simulink model "pmsm_ctrl"  (R2018a)
settings: Solver=FixedStepDiscrete  StartTime=0.0  StopTime=3  FixedStep=FastTsample / 10.  RelTol=1e-3  EnableMultiTasking=on
model workspace (MATLAB code in the model file):
  | cmdLim = Simulink.Parameter;
  | cmdLim.Value = 15;
  | cmdLim.Description = 'Limit for controlling the maximum surface command angle.';
  | cmdLim.Min = 0;
  | cmdLim.Max = 90;
  | cmdLim.DocUnits = 'deg';
  | 
  | dispGain = Simulink.Parameter;
  | dispGain.Value = 0.75;
  | dispGain.Description = 'Gain applied to the displacement error.';
  | dispGain.Min = 0;
  | dispGain.Max = [];
  | dispGain.DocUnits = 'deg/sec/deg';
  | 
  | dispLim = Simulink.Parameter;
  | dispLim.Value = 30;
  | dispLim.Description = 'Limit for controlling the maximum commanded angle.';
  | dispLim.Min = 0;
  | dispLim.Max = 180;
  | dispLim.DocUnits = 'deg';
  | 
  | intGain = Simulink.Parameter;
  | intGain.Value = 0.5;
  | intGain.Description = 'Gain applied to the integral error.';
  | intGain.Min = 0;
  | intGain.Max = [];
  | intGain.DocUnits = 'deg/sec/deg/sec';
  | 
  | intLim = Simulink.Parameter;
  | intLim.Value = 5;
  | intLim.Description = 'Limit for controlling the maximum commanded angle.';
  | intLim.Min = 0;
  | intLim.Max = 90;
  | intLim.DocUnits = 'deg';
  | 
  | rateGain = Simulink.Parameter;
  | rateGain.Value = 2;
  | rateGain.Description = 'Gain applied to the rate error.';
  | rateGain.Min = 0;
  | rateGain.Max = [];
  | rateGain.DocUnits = 'deg/deg/sec';
  | 
  | rateLim = Simulink.Parameter;
  | rateLim.Value = 6;
  | rateLim.Description = 'Limit for controlling the maximum commanded angle.';
  | rateLim.Min = 0;
  | rateLim.Max = 180;
  | rateLim.DocUnits = 'deg/sec';
  | 
  | hdgGain = Simulink.Parameter;
  | hdgGain.Value = 0.015;
undefined symbols (not defined in the file): CalMgrSt_T, Cfg_AnglOfsCalPwmDuty, Cfg_AutoCalEnbl, Cfg_EnblDynComp, Cfg_EnblTrajPlan, Cfg_EncCnts, Cfg_EncOfsCalPwmDuty, Cfg_IfbkCtrlBW, Cfg_IndCalPwmDuty, Cfg_Ls, Cfg_MFlux, Cfg_MtrJm, Cfg_MtrKf, Cfg_MtrKtrq, Cfg_PolePairs, Cfg_ResCalPwmDuty, Cfg_Rs, Cfg_SpdCtrlBW, Cfg_SpdSnsEnbl, Cfg_StepToEncCnts, Cfg_UseObsPosEst, Cfg_VBus, DiscIntNeverNeededParam, DistObs_J, EncCntsToRads, MtrCtrlCal_T, MtrCtrlMd, MtrCtrlMd_T, MtrParams, TsFast, TsMain
libraries: ctrl_lib x13, simulink x10, adrc_lib x2, peTransforms x1
(part 1 of 2)
settings Model: RequirementInfo={} %GIDa_fe9045fd_0412_4b6e_8206_617cc20e6fde  FPTRunName=Active  Creator=elrobotista  LastModifiedBy=elrobotista
settings SolverCC: MinimalZcImpactIntegration=on
settings DataIOCC: SaveFormat=StructureWithTime  SaveOutput=off  SignalLogging=off  DSMLogging=off  SaveTime=off
settings OptimizationCC: DefaultParameterBehavior=Inlined  UseDivisionForNetSlopeComputation=on  UseFloatMulNetSlope=on  DefaultUnderspecifiedDataType=single  UseSpecifiedMinMax=on  InlineInvariantSignals=on  StrengthReduction=on  PassReuseOutputArgsAs=Individual arguments  ZeroExternalMemoryAtStartup=off  ZeroInternalMemoryAtStartup=off  NoFixptDivByZeroProtection=on  EfficientFloat2IntCast=on  LifeSpan=1  OptimizeBlockOrder=speed  OptimizationPriority=Speed  OptimizationCustomize=off  LabelGuidedReuse=on
settings DebuggingCC: AllowSymbolicDim=off  StrictBusMsg=ErrorOnBusTreatedAsVector  SFUnexpectedBacktrackingDiag=warning  SFNoUnconditionalDefaultTransitionDiag=warning  SFExecutionAtInitializationDiag=none
settings HardwareCC: ProdBitPerPointer=32  ProdBitPerSizeT=32  ProdBitPerPtrDiffT=32  ProdLargestAtomicInteger=Long  ProdLargestAtomicFloat=Double  ProdWordSize=32  ProdHWDeviceType=ARM Compatible->ARM Cortex
settings ModelReferenceCC: ModelReferenceNumInstancesAllowed=Single
settings SFSimCC: MATLABDynamicMemAlloc=off
settings RTWCC: SystemTargetFile=ert.tlc  GenCodeOnly=on  PackageGeneratedCodeAndArtifacts=on  TemplateMakefile=ert_default_tmf  GenerateReport=on  BuildConfiguration=Faster Runs  IncludeHyperlinkInReport=on  LaunchReport=on  GenerateTraceInfo=on  GenerateTraceReport=on  GenerateTraceReportSl=on  GenerateTraceReportSf=on  GenerateTraceReportEml=on  GenerateCodeMetricsReport=on
settings CodeAppCC: ForceParamTrailComments=on  IgnoreCustomStorageClasses=off  OperatorAnnotations=on  SimulinkDataObjDesc=on  SFDataObjDesc=on  CustomSymbolStrGlobalVar=rt$N$M  CustomSymbolStrType=$N$M  CustomSymbolStrFcn=$N$M$F  CustomSymbolStrMacro=$N$M  InsertBlockDesc=on  EnableCustomComments=on  ReqsInCode=on
settings ERTTargetCC: CodeReplacementLibrary=ARM Cortex-M (Optimized)  MultiwordLength=2048  GenerateFullHeader=off  IncludeMdlTerminateFcn=off  SuppressErrorStatus=on  ERTCustomFileBanners=off  SupportAbsoluteTime=off  MultiInstanceERTCode=on  CodeInterfacePackaging=Reusable function  SupportNonFinite=off  SupportComplex=off  RemoveDisableFunc=on  InlinedParameterPlacement=NonHierarchical  MultiInstanceErrorCode=Warning  ERTCustomFileTemplate=example_file_process.tlc
settings ConfigComp: CovScope=ReferencedModels  CovSaveName=covdata_rollAP  CovMetricSettings=dcmtrwe  CovHTMLOptions=-sRT=1 -aTS=1 -bRG=1 -bTC=1 -hTR=1 -nFC=0 -scm=1 -bcm=1 -xEv=0  CovSaveCumulativeToWorkspaceVar=on  CovSaveSingleToWorkspaceVar=on  CovCumulativeVarName=covCumulativeData_rollAP  CovReportOnPause=off  CovExternalEMLEnable=off  CovSFcnEnable=off

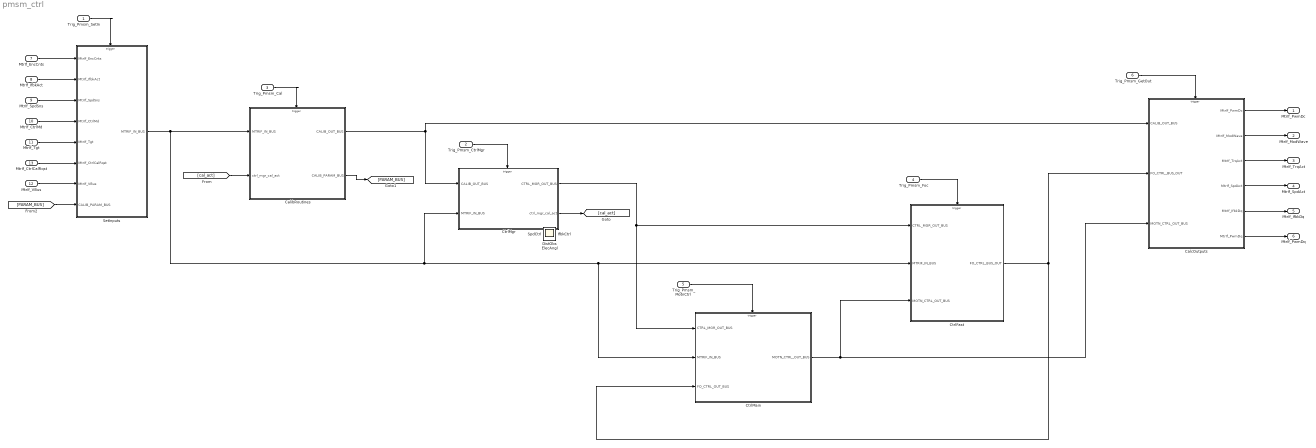
== system pmsm_ctrl ==
  Trig_Pmsm_SetIn : Inport  OutDataTypeStr=double  OutputFunctionCall=on
  Trig_Pmsm_CtrlMgr : Inport  Port=2  OutDataTypeStr=double  OutputFunctionCall=on
  Trig_Pmsm_Cal : Inport  Port=3  OutDataTypeStr=double  OutputFunctionCall=on
  Trig_Pmsm_Foc : Inport  Port=4  OutDataTypeStr=double  OutputFunctionCall=on
  Trig_Pmsm_MotnCtrl : Inport  Port=5  OutDataTypeStr=double  OutputFunctionCall=on
  Trig_Pmsm_GetOut : Inport  Port=6  OutDataTypeStr=double  OutputFunctionCall=on
  MtrIf_EncCnts : Inport  Port=7
      settings: AttributesFormatString=%<OutDataTypeStr>
  MtrIf_IfbkAct : Inport  Port=8  PortDimensions=3
  MtrIf_SpdSns : Inport  Port=9
  MtrIf_CtrlMd : Inport  Port=10
  MtrIf_Tgt : Inport  Port=11
  MtrIf_VBus : Inport  Port=12
      settings: AttributesFormatString=%<OutDataTypeStr>
  MtrIf_CtrlCalRqst : Inport  Port=13
      settings: AttributesFormatString=%<OutDataTypeStr>
  CalcOutputs : Subsystem
  CalibRoutines : Subsystem
  CtrlFast : Subsystem  TreatAsAtomicUnit=on  RTWFcnName=foo
  CtrlMain : Subsystem  TreatAsAtomicUnit=on  RTWFcnName=foo
      settings: FunctionInterfaceSpec=Allow arguments
  CtrlMgr : Subsystem
  SetInputs : Subsystem
  MtrIf_PwmDc : Outport
  MtrIf_ModWave : Outport  Port=2
  MtrIf_TrqAct : Outport  Port=3
  MtrIf_SpdAct : Outport  Port=4
  MtrIf_IfbkDq : Outport  Port=5
  MtrIf_PwmDq : Outport  Port=6
  DistObs : Scope
  ElecAngl : Scope
  IfbkCtrl : Scope
  SpdCtrl : Scope
  wires:
  Trig_Pmsm_Foc/1 -> CtrlFast/Trigger
  Trig_Pmsm_MotnCtrl/1 -> CtrlMain/Trigger
  CtrlMain/1(MOTN_CTRL_OUT_BUS) -> CalcOutputs/3(MOTN_CTRL_OUT_BUS), CtrlFast/3(MOTN_CTRL_OUT_BUS)
  Trig_Pmsm_CtrlMgr/1 -> CtrlMgr/Trigger
  Trig_Pmsm_GetOut/1 -> CalcOutputs/Trigger
  Trig_Pmsm_Cal/1 -> CalibRoutines/Trigger
  Trig_Pmsm_SetIn/1 -> SetInputs/Trigger
  MtrIf_EncCnts/1 -> SetInputs/1(MtrIf_EncCnts)
  MtrIf_IfbkAct/1 -> SetInputs/2(MtrIf_IfbkAct)
  MtrIf_SpdSns/1 -> SetInputs/3(MtrIf_SpdSns)
  MtrIf_CtrlMd/1 -> SetInputs/4(MtrIf_CtrlMd)
  MtrIf_Tgt/1 -> SetInputs/5(MtrIf_Tgt)
  SetInputs/1(MTRIF_IN_BUS) -> CalibRoutines/1(MTRIF_IN_BUS), CtrlMain/2(MTRIF_IN_BUS), CtrlFast/2(MTRIF_IN_BUS), CtrlMgr/2(MTRIF_IN_BUS)
  CtrlFast/1(FO_CTRL_BUS_OUT) -> CalcOutputs/2(FO_CTRL_BUS_OUT), CtrlMain/3(FO_CTRL_OUT_BUS)
  CalibRoutines/1(CALIB_OUT_BUS) -> CalcOutputs/1(CALIB_OUT_BUS), CtrlMgr/1(CALIB_OUT_BUS)
  CalcOutputs/1(MtrIf_PwmDc) -> MtrIf_PwmDc/1
  CalcOutputs/2(MtrIf_ModWave) -> MtrIf_ModWave/1
  CalcOutputs/3(MtrIf_TrqAct) -> MtrIf_TrqAct/1
  CalcOutputs/4(MtrIf_SpdAct) -> MtrIf_SpdAct/1
  CtrlMgr/1(CTRL_MGR_OUT_BUS) -> CtrlFast/1(CTRL_MGR_OUT_BUS), CtrlMain/1(CTRL_MGR_OUT_BUS)
  MtrIf_CtrlCalRqst/1 -> SetInputs/6(MtrIf_CtrlCalRqst)
  CtrlMgr/2(ctrl_mgr_cal_act) -> [cal_act]
  [cal_act] -> CalibRoutines/2(ctrl_mgr_cal_act)
  CalibRoutines/2(CALIB_PARAM_BUS) -> [PARAM_BUS]
  [PARAM_BUS] -> SetInputs/8(CALIB_PARAM_BUS)
  CalcOutputs/5(MtrIf_IfbkDq) -> MtrIf_IfbkDq/1
  CalcOutputs/6(MtrIf_PwmDq) -> MtrIf_PwmDq/1
  MtrIf_VBus/1 -> SetInputs/7(MtrIf_VBus)

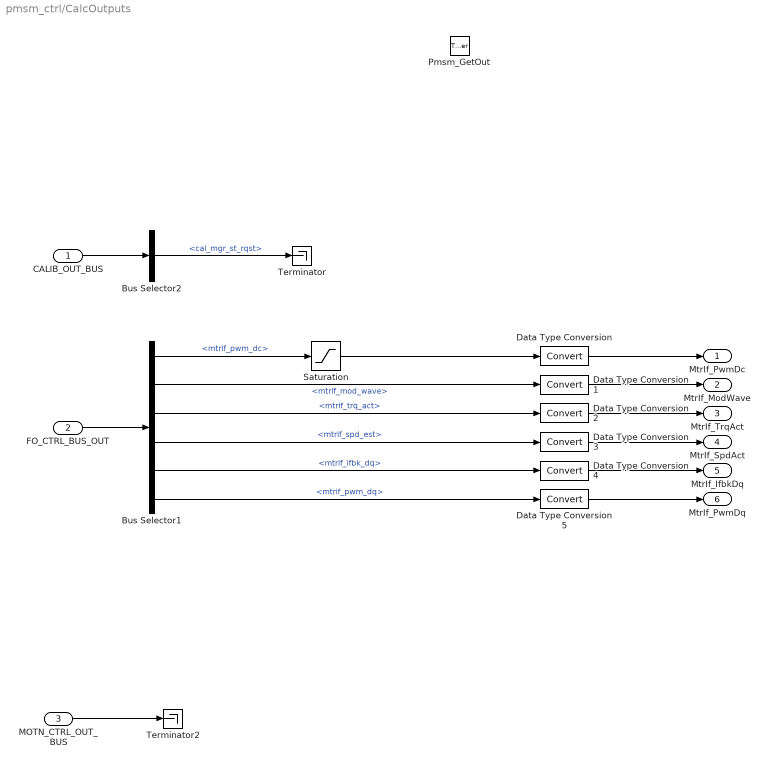
== system pmsm_ctrl/CalcOutputs ==
  CALIB_OUT_BUS : Inport  OutDataTypeStr=Bus: Calib_OutType
  FO_CTRL_BUS_OUT : Inport  Port=2  OutDataTypeStr=Bus: FoCtrl_OutType
  MOTN_CTRL_OUT_BUS : Inport  Port=3  OutDataTypeStr=Bus: MotnCtrl_OutType
  Pmsm_GetOut : TriggerPort  TriggerType=function-call  VariantControl=Variant  SampleTime=-1
  Bus Selector1 : BusSelector  OutputSignals=mtrif_pwm_dc,mtrif_mod_wave,mtrif_trq_act,mtrif_spd_est,mtrif_ifbk_dq,mtrif_pwm_dq
  Bus Selector2 : BusSelector  OutputSignals=cal_mgr_st_rqst
  Data Type Conversion{,1..5} (6 alike) : DataTypeConversion
  Saturation : Saturate  UpperLimit=1.  LowerLimit=0.
  Terminator : Terminator
  Terminator2 : Terminator
  MtrIf_PwmDc : Outport
  MtrIf_ModWave : Outport  Port=2
  MtrIf_TrqAct : Outport  Port=3
  MtrIf_SpdAct : Outport  Port=4
  MtrIf_IfbkDq : Outport  Port=5
  MtrIf_PwmDq : Outport  Port=6
  wires:
  CALIB_OUT_BUS/1 -> Bus Selector2/1
  FO_CTRL_BUS_OUT/1 -> Bus Selector1/1
  MOTN_CTRL_OUT_BUS/1 -> Terminator2/1
  Bus Selector1/3 -> Data Type Conversion2/1  "<mtrif_trq_act>"
  Bus Selector1/4 -> Data Type Conversion3/1  "<mtrif_spd_est>"
  Data Type Conversion/1 -> MtrIf_PwmDc/1
  Data Type Conversion1/1 -> MtrIf_ModWave/1
  Data Type Conversion2/1 -> MtrIf_TrqAct/1
  Data Type Conversion3/1 -> MtrIf_SpdAct/1
  Saturation/1 -> Data Type Conversion/1
  Bus Selector1/1 -> Saturation/1  "<mtrif_pwm_dc>"
  Bus Selector1/2 -> Data Type Conversion1/1  "<mtrif_mod_wave>"
  Bus Selector2/1 -> Terminator/1  "<cal_mgr_st_rqst>"
  Data Type Conversion4/1 -> MtrIf_IfbkDq/1
  Bus Selector1/5 -> Data Type Conversion4/1  "<mtrif_ifbk_dq>"
  Data Type Conversion5/1 -> MtrIf_PwmDq/1
  Bus Selector1/6 -> Data Type Conversion5/1  "<mtrif_pwm_dq>"

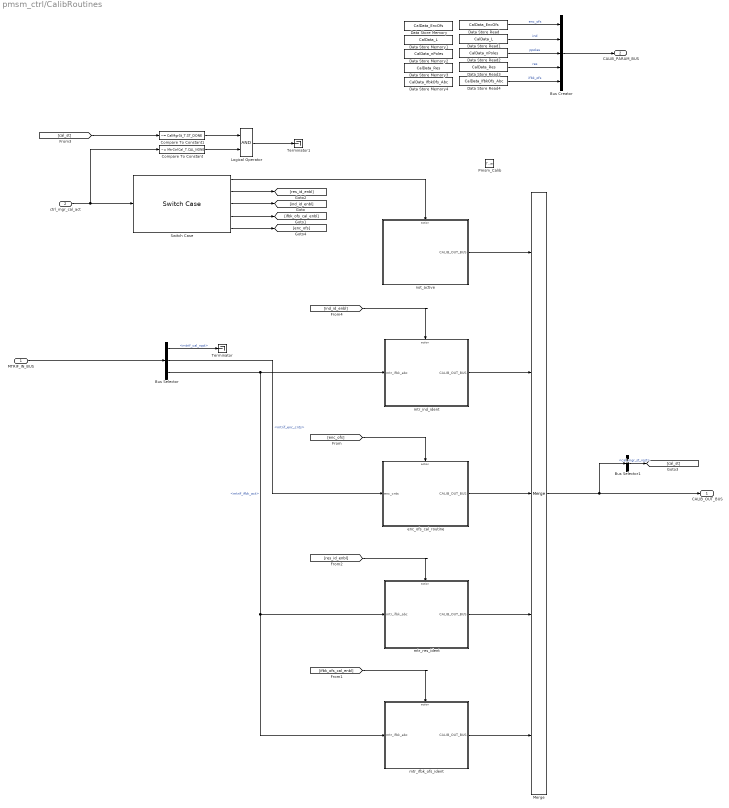
== system pmsm_ctrl/CalibRoutines ==
  MTRIF_IN_BUS : Inport  OutDataTypeStr=Bus: MtrIf_InType
  ctrl_mgr_cal_act : Inport  Port=2
  Pmsm_Calib : TriggerPort  TriggerType=function-call  VariantControl=Variant  SampleTime=-1
  Bus Creator : BusCreator  Inputs=5  OutDataTypeStr=Bus: Calib_ParamType  NonVirtualBus=on
  Bus Selector : BusSelector  OutputSignals=mtrif_cal_rqst,mtrif_enc_cnts,mtrif_ifbk_act
  Bus Selector1 : BusSelector  OutputSignals=cal_mgr_st_rqst
  Compare To Constant : simulink/Logic and Bit Operations/Compare To Constant  relop=~=  const=MtrCtrlCal_T.CAL_NONE  OutDataTypeStr=boolean
  Compare To Constant1 : simulink/Logic and Bit Operations/Compare To Constant  relop=~=  const=CalMgrSt_T.ST_DONE  OutDataTypeStr=boolean
  Data Store Memory : DataStoreMemory  DataStoreName=CalData_EncOfs  ReadBeforeWriteMsg=warning  WriteAfterWriteMsg=warning  WriteAfterReadMsg=warning  ShareAcrossModelInstances=on  ShowAdditionalParam=off  OutDataTypeStr=int32  Dimensions=1
      settings: RTWStateStorageClass=ExportedGlobal
  Data Store Memory1 : DataStoreMemory  DataStoreName=CalData_L  ReadBeforeWriteMsg=warning  WriteAfterWriteMsg=warning  WriteAfterReadMsg=warning  InitialValue=-1.  ShareAcrossModelInstances=on  ShowAdditionalParam=off  OutDataTypeStr=single  Dimensions=1
      settings: RTWStateStorageClass=ExportedGlobal
  Data Store Memory2 : DataStoreMemory  DataStoreName=CalData_nPoles  ReadBeforeWriteMsg=warning  WriteAfterWriteMsg=warning  WriteAfterReadMsg=warning  ShareAcrossModelInstances=on  ShowAdditionalParam=off  OutDataTypeStr=int32  Dimensions=1
      settings: RTWStateStorageClass=ExportedGlobal
  Data Store Memory3 : DataStoreMemory  DataStoreName=CalData_Res  ReadBeforeWriteMsg=warning  WriteAfterWriteMsg=warning  WriteAfterReadMsg=warning  InitialValue=-1.  ShareAcrossModelInstances=on  ShowAdditionalParam=off  OutDataTypeStr=single  Dimensions=1
      settings: RTWStateStorageClass=ExportedGlobal
  Data Store Memory4 : DataStoreMemory  DataStoreName=CalData_IfbkOfs_Abc  ReadBeforeWriteMsg=warning  WriteAfterWriteMsg=warning  WriteAfterReadMsg=warning  InitialValue=[0., 0., 0.]  ShareAcrossModelInstances=on  ShowAdditionalParam=off  OutDataTypeStr=single  Dimensions=3
      settings: RTWStateStorageClass=ExportedGlobal
  Data Store Read : DataStoreRead  DataStoreName=CalData_EncOfs
  Data Store Read1 : DataStoreRead  DataStoreName=CalData_L
  Data Store Read2 : DataStoreRead  DataStoreName=CalData_nPoles
  Data Store Read3 : DataStoreRead  DataStoreName=CalData_Res
  Data Store Read4 : DataStoreRead  DataStoreName=CalData_IfbkOfs_Abc
  Logical Operator : Logic  AllPortsSameDT=off  OutDataTypeStr=boolean
  Merge : Merge  Inputs=5
  Switch Case : SwitchCase  CaseConditions={MtrCtrlCal_T.CAL_NONE, MtrCtrlCal_T.CAL_RES_ID, MtrCtrlCal_T.CAL_IND_ID, MtrCtrlCal_T.CAL_IFBK_OFS, MtrCtrlCal_T.CAL_ENC_OFS}  ShowDefaultCase=off
  Terminator : Terminator
  Terminator1 : Terminator
  enc_ofs_cal_routine : Subsystem
  mtr_ifbk_ofs_ident : Subsystem
  mtr_ind_ident : Subsystem
  mtr_res_ident : Subsystem
  not_active : Subsystem
  CALIB_OUT_BUS : Outport  OutDataTypeStr=Bus: Calib_OutType
  CALIB_PARAM_BUS : Outport  Port=2  OutDataTypeStr=Bus: Calib_ParamType
  wires:
  MTRIF_IN_BUS/1 -> Bus Selector/1
  Bus Selector/2 -> enc_ofs_cal_routine/1(enc_cnts)  "<mtrif_enc_cnts>"
  Bus Selector/1 -> Terminator/1  "<mtrif_cal_rqst>"
  Merge/1 -> Bus Selector1/1, CALIB_OUT_BUS/1
  Bus Selector/3 -> mtr_ifbk_ofs_ident/1(mtr_ifbk_abc), mtr_res_ident/1(mtr_ifbk_abc), mtr_ind_ident/1(mtr_ifbk_abc)  "<mtrif_ifbk_act>"
  Switch Case/2 -> [res_id_enbl]
  [res_id_enbl] -> mtr_res_ident/Action
  Switch Case/3 -> [ind_id_enbl]
  [ifbk_ofs_cal_enbl] -> mtr_ifbk_ofs_ident/Action
  Switch Case/4 -> [ifbk_ofs_cal_enbl]
  [enc_ofs] -> enc_ofs_cal_routine/Action
  not_active/1(CALIB_OUT_BUS) -> Merge/1
  Switch Case/1 -> not_active/Action
  ctrl_mgr_cal_act/1 -> Switch Case/1, Compare To Constant/1
  Compare To Constant/1 -> Logical Operator/2
  Logical Operator/1 -> Terminator1/1
  Compare To Constant1/1 -> Logical Operator/1
  Bus Selector1/1 -> [cal_st]  "<cal_mgr_st_rqst>"
  [cal_st] -> Compare To Constant1/1
  Switch Case/5 -> [enc_ofs]
  enc_ofs_cal_routine/1(CALIB_OUT_BUS) -> Merge/3
  mtr_res_ident/1(CALIB_OUT_BUS) -> Merge/4
  mtr_ifbk_ofs_ident/1(CALIB_OUT_BUS) -> Merge/5
  mtr_ind_ident/1(CALIB_OUT_BUS) -> Merge/2
  [ind_id_enbl] -> mtr_ind_ident/Action
  Bus Creator/1 -> CALIB_PARAM_BUS/1
  Data Store Read/1 -> Bus Creator/1  "enc_ofs"
  Data Store Read1/1 -> Bus Creator/2  "ind"
  Data Store Read2/1 -> Bus Creator/3  "ppoles"
  Data Store Read3/1 -> Bus Creator/4  "res"
  Data Store Read4/1 -> Bus Creator/5  "ifbk_ofs"

== system pmsm_ctrl/CtrlFast ==
  CTRL_MGR_OUT_BUS : Inport  OutDataTypeStr=Bus: CtrlMgr_OutType
  MTRIF_IN_BUS : Inport  Port=2  OutDataTypeStr=Bus: MtrIf_InType
  MOTN_CTRL_OUT_BUS : Inport  Port=3
  Pmsm_Foc : TriggerPort  TriggerType=function-call  VariantControl=Variant  SampleTime=-1
  Bus Creator : BusCreator  Inputs=7
  Bus Selector : BusSelector  OutputSignals=mtrif_enc_cnts,mtrif_ifbk_act,mtrif_spd_sns
  Field_Oriented_Controller : Subsystem
  det_ctrl_tgt : Subsystem
  FO_CTRL_BUS_OUT : Outport  OutDataTypeStr=Bus: FoCtrl_OutType  InitialOutput=0
  wires:
  MTRIF_IN_BUS/1 -> Bus Selector/1
  Field_Oriented_Controller/1(MtrIf_ModWave) -> Bus Creator/1  "mtrif_mod_wave"
  Field_Oriented_Controller/2(MtrIf_SpdOut) -> Bus Creator/2  "mtrif_spd_est"
  Field_Oriented_Controller/3(MtrIf_PwmDc) -> Bus Creator/3  "mtrif_pwm_dc"
  Field_Oriented_Controller/4(MtrIf_TrqAct) -> Bus Creator/4  "mtrif_trq_act"
  Field_Oriented_Controller/5(obs_enc_cnts) -> Bus Creator/5  "obs_enc_cnts"
  Bus Selector/1 -> Field_Oriented_Controller/1(MtrIf_EncCnts)  "<mtrif_enc_cnts>"
  Bus Selector/2 -> Field_Oriented_Controller/2(MtrIf_IfbkAct)  "<mtrif_ifbk_act>"
  Bus Selector/3 -> Field_Oriented_Controller/3(MtrIf_SpdSns)  "<mtrif_spd_sns>"
  Bus Creator/1 -> FO_CTRL_BUS_OUT/1
  CTRL_MGR_OUT_BUS/1 -> Field_Oriented_Controller/4(CTRL_MGR_OUT_BUS), det_ctrl_tgt/1(CTRL_MGR_OUT_BUS)
  MOTN_CTRL_OUT_BUS/1 -> det_ctrl_tgt/2(MOTN_CTRL_OUT_BUS)
  det_ctrl_tgt/1(ctrl_tgt) -> Field_Oriented_Controller/5(ctrl_tgt)
  Field_Oriented_Controller/6(MtrIf_IfbkDq) -> Bus Creator/6  "mtrif_ifbk_dq"
  Field_Oriented_Controller/7(MtrIf_PwmDq) -> Bus Creator/7  "mtrif_pwm_dq"

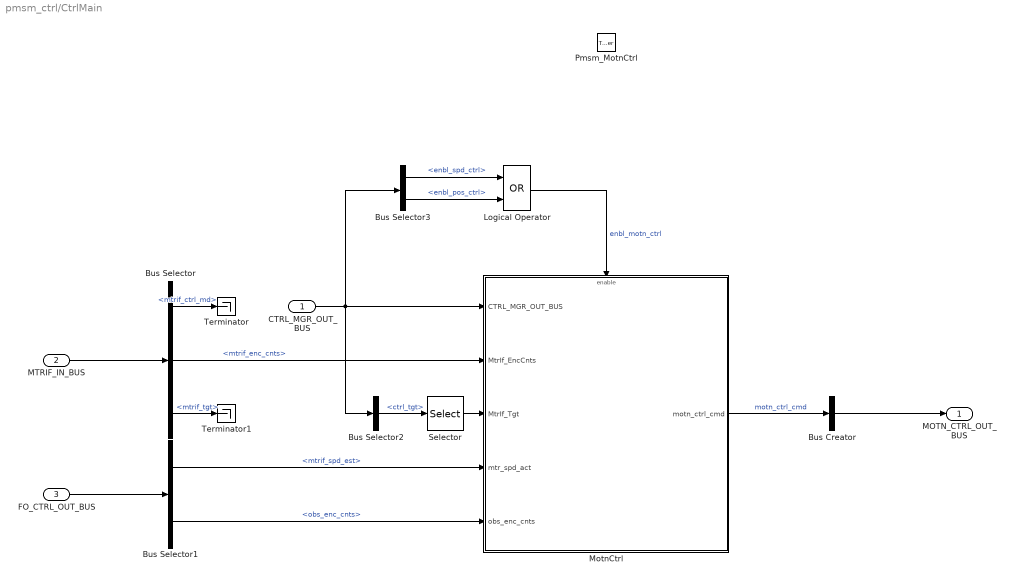
== system pmsm_ctrl/CtrlMain ==
  CTRL_MGR_OUT_BUS : Inport  OutDataTypeStr=Bus: CtrlMgr_OutType
  MTRIF_IN_BUS : Inport  Port=2  OutDataTypeStr=Bus: MtrIf_InType
  FO_CTRL_OUT_BUS : Inport  Port=3  OutDataTypeStr=Bus: FoCtrl_OutType
  Pmsm_MotnCtrl : TriggerPort  TriggerType=function-call  VariantControl=Variant  SampleTime=-1
  Bus Creator : BusCreator  Inputs=1  OutDataTypeStr=Bus: MotnCtrl_OutType  NonVirtualBus=on
  Bus Selector : BusSelector  OutputSignals=mtrif_ctrl_md,mtrif_enc_cnts,mtrif_tgt
  Bus Selector1 : BusSelector  OutputSignals=mtrif_spd_est,obs_enc_cnts
  Bus Selector2 : BusSelector  OutputSignals=ctrl_tgt
  Bus Selector3 : BusSelector  OutputSignals=enbl_ctrl_flags.enbl_spd_ctrl,enbl_ctrl_flags.enbl_pos_ctrl
  Logical Operator : Logic  Operator=OR  AllPortsSameDT=off  OutDataTypeStr=boolean
  MotnCtrl : Subsystem
  Selector : Selector  InputPortWidth=3  IndexOptions=Index vector (dialog)  Indices=[1]  OutputSizes=1
  Terminator : Terminator
  Terminator1 : Terminator
  MOTN_CTRL_OUT_BUS : Outport  OutDataTypeStr=Bus: MotnCtrl_OutType  InitialOutput=0
  wires:
  MTRIF_IN_BUS/1 -> Bus Selector/1
  Bus Selector/1 -> Terminator/1  "<mtrif_ctrl_md>"
  Bus Selector/2 -> MotnCtrl/2(MtrIf_EncCnts)  "<mtrif_enc_cnts>"
  Bus Creator/1 -> MOTN_CTRL_OUT_BUS/1
  MotnCtrl/1(motn_ctrl_cmd) -> Bus Creator/1  "motn_ctrl_cmd"
  FO_CTRL_OUT_BUS/1 -> Bus Selector1/1
  Bus Selector1/1 -> MotnCtrl/4(mtr_spd_act)  "<mtrif_spd_est>"
  Bus Selector1/2 -> MotnCtrl/5(obs_enc_cnts)  "<obs_enc_cnts>"
  CTRL_MGR_OUT_BUS/1 -> Bus Selector3/1, MotnCtrl/1(CTRL_MGR_OUT_BUS), Bus Selector2/1
  Bus Selector2/1 -> Selector/1  "<ctrl_tgt>"
  Bus Selector/3 -> Terminator1/1  "<mtrif_tgt>"
  Bus Selector3/1 -> Logical Operator/1  "<enbl_spd_ctrl>"
  Bus Selector3/2 -> Logical Operator/2  "<enbl_pos_ctrl>"
  Logical Operator/1 -> MotnCtrl/Enable  "enbl_motn_ctrl"
  Selector/1 -> MotnCtrl/3(MtrIf_Tgt)

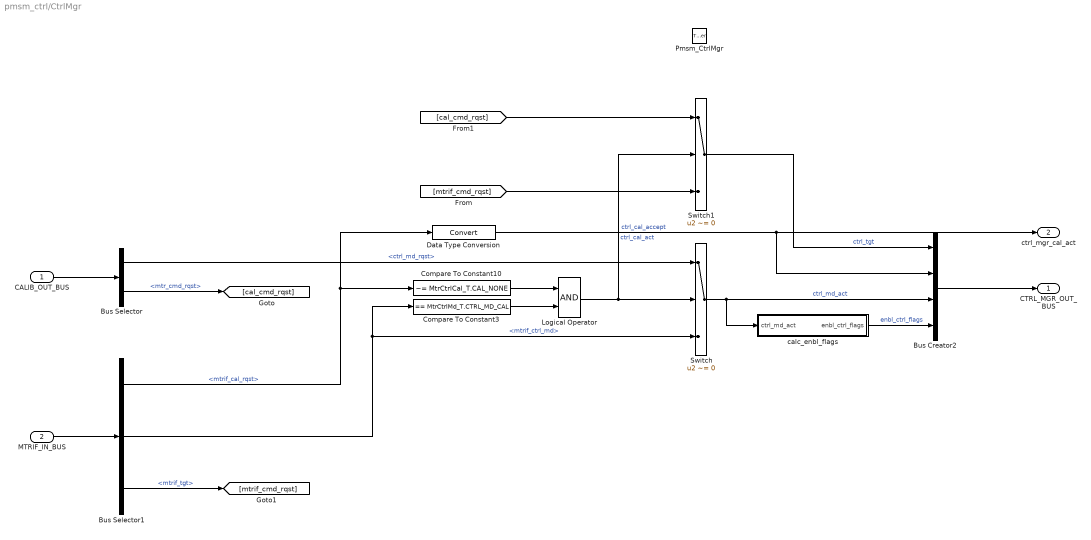
== system pmsm_ctrl/CtrlMgr ==
  CALIB_OUT_BUS : Inport  OutDataTypeStr=Bus: Calib_OutType
  MTRIF_IN_BUS : Inport  Port=2  OutDataTypeStr=Bus: MtrIf_InType
  Pmsm_CtrlMgr : TriggerPort  TriggerType=function-call  VariantControl=Variant  SampleTime=-1
  Bus Creator2 : BusCreator  Inputs=4  OutDataTypeStr=Bus: CtrlMgr_OutType  NonVirtualBus=on
  Bus Selector : BusSelector  OutputSignals=ctrl_md_rqst,mtr_cmd_rqst
  Bus Selector1 : BusSelector  OutputSignals=mtrif_cal_rqst,mtrif_ctrl_md,mtrif_tgt
  Compare To Constant10 : simulink/Logic and Bit Operations/Compare To Constant  relop=~=  const=MtrCtrlCal_T.CAL_NONE  OutDataTypeStr=boolean
  Compare To Constant3 : simulink/Logic and Bit Operations/Compare To Constant  relop===  const=MtrCtrlMd_T.CTRL_MD_CAL  OutDataTypeStr=boolean
  Data Type Conversion : DataTypeConversion
  Logical Operator : Logic  AllPortsSameDT=off  OutDataTypeStr=boolean
  Switch : Switch  Criteria=u2 ~= 0
  Switch1 : Switch  Criteria=u2 ~= 0
  calc_enbl_flags : Subsystem
  CTRL_MGR_OUT_BUS : Outport  OutDataTypeStr=Bus: CtrlMgr_OutType
  ctrl_mgr_cal_act : Outport  Port=2
  wires:
  CALIB_OUT_BUS/1 -> Bus Selector/1
  MTRIF_IN_BUS/1 -> Bus Selector1/1
  Bus Selector1/2 -> Switch/3, Compare To Constant3/1  "<mtrif_ctrl_md>"
  Bus Selector1/1 -> Data Type Conversion/1, Compare To Constant10/1  "<mtrif_cal_rqst>"
  Compare To Constant10/1 -> Logical Operator/1
  Logical Operator/1 -> Switch/2, Switch1/2  "ctrl_cal_accept"
  Compare To Constant3/1 -> Logical Operator/2
  Bus Creator2/1 -> CTRL_MGR_OUT_BUS/1
  Switch/1 -> calc_enbl_flags/1(ctrl_md_act), Bus Creator2/3  "ctrl_md_act"
  Bus Selector/1 -> Switch/1  "<ctrl_md_rqst>"
  Data Type Conversion/1 -> ctrl_mgr_cal_act/1, Bus Creator2/2  "ctrl_cal_act"
  Bus Selector/2 -> [cal_cmd_rqst]  "<mtr_cmd_rqst>"
  [cal_cmd_rqst] -> Switch1/1
  Switch1/1 -> Bus Creator2/1  "ctrl_tgt"
  [mtrif_cmd_rqst] -> Switch1/3
  Bus Selector1/3 -> [mtrif_cmd_rqst]  "<mtrif_tgt>"
  calc_enbl_flags/1(enbl_ctrl_flags) -> Bus Creator2/4  "enbl_ctrl_flags"

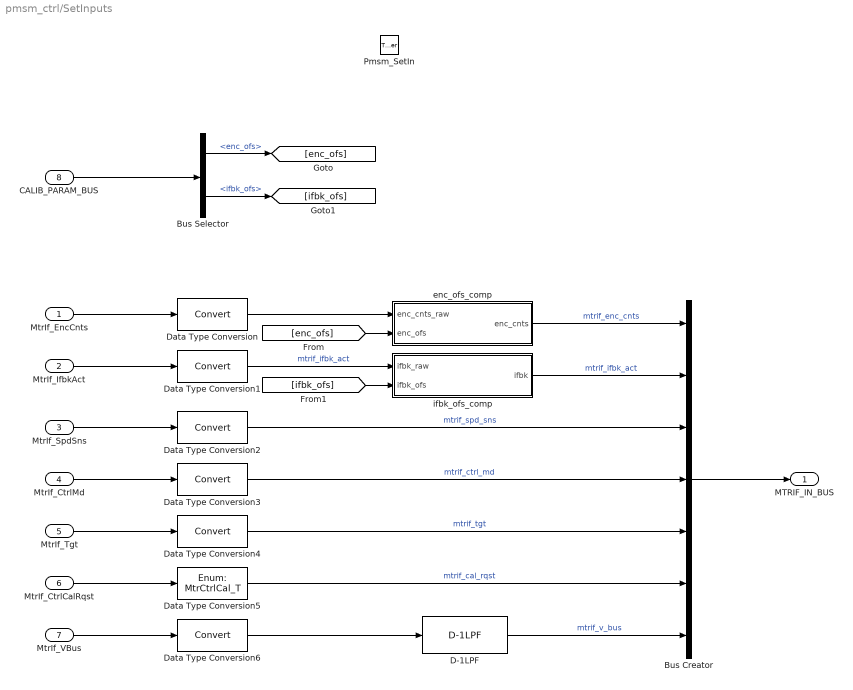
== system pmsm_ctrl/SetInputs ==
  MtrIf_EncCnts : Inport  OutDataTypeStr=int32
      settings: AttributesFormatString=%<OutDataTypeStr>
  MtrIf_IfbkAct : Inport  Port=2  PortDimensions=3
  MtrIf_SpdSns : Inport  Port=3
  MtrIf_CtrlMd : Inport  Port=4  OutDataTypeStr=Enum: MtrCtrlMd_T
  MtrIf_Tgt : Inport  Port=5
  MtrIf_CtrlCalRqst : Inport  Port=6
      settings: AttributesFormatString=%<OutDataTypeStr>
  MtrIf_VBus : Inport  Port=7
      settings: AttributesFormatString=%<OutDataTypeStr>
  CALIB_PARAM_BUS : Inport  Port=8  OutDataTypeStr=Bus: Calib_ParamType
      settings: AttributesFormatString=%<OutDataTypeStr>
  Pmsm_SetIn : TriggerPort  TriggerType=function-call  VariantControl=Variant  SampleTime=-1
  Bus Creator : BusCreator  Inputs=7  OutDataTypeStr=Bus: MtrIf_InType  NonVirtualBus=on
  Bus Selector : BusSelector  OutputSignals=enc_ofs,ifbk_ofs
  D-1LPF : ctrl_lib/D-1LPF  k_filt=0.01/ (0.01 + TsFast)
  Data Type Conversion{,1..4,6} (6 alike) : DataTypeConversion
  Data Type Conversion5 : DataTypeConversion  OutDataTypeStr=Enum: MtrCtrlCal_T
  enc_ofs_comp : Subsystem
  ifbk_ofs_comp : Subsystem
  MTRIF_IN_BUS : Outport  OutDataTypeStr=Bus: MtrIf_InType
  wires:
  MtrIf_EncCnts/1 -> Data Type Conversion/1
  MtrIf_IfbkAct/1 -> Data Type Conversion1/1
  MtrIf_SpdSns/1 -> Data Type Conversion2/1
  MtrIf_CtrlMd/1 -> Data Type Conversion3/1
  MtrIf_Tgt/1 -> Data Type Conversion4/1
  MtrIf_CtrlCalRqst/1 -> Data Type Conversion5/1
  Data Type Conversion4/1 -> Bus Creator/5  "mtrif_tgt"
  Data Type Conversion5/1 -> Bus Creator/6  "mtrif_cal_rqst"
  Data Type Conversion3/1 -> Bus Creator/4  "mtrif_ctrl_md"
  enc_ofs_comp/1(enc_cnts) -> Bus Creator/1  "mtrif_enc_cnts"
  Data Type Conversion1/1 -> ifbk_ofs_comp/1(ifbk_raw)  "mtrif_ifbk_act"
  Data Type Conversion2/1 -> Bus Creator/3  "mtrif_spd_sns"
  Bus Creator/1 -> MTRIF_IN_BUS/1
  Data Type Conversion/1 -> enc_ofs_comp/1(enc_cnts_raw)
  CALIB_PARAM_BUS/1 -> Bus Selector/1
  Bus Selector/1 -> [enc_ofs]  "<enc_ofs>"
  [enc_ofs] -> enc_ofs_comp/2("enc_ofs ")
  ifbk_ofs_comp/1(ifbk) -> Bus Creator/2  "mtrif_ifbk_act"
  Bus Selector/2 -> [ifbk_ofs]  "<ifbk_ofs>"
  [ifbk_ofs] -> ifbk_ofs_comp/2("ifbk_ofs ")
  Data Type Conversion6/1 -> D-1LPF/1
  MtrIf_VBus/1 -> Data Type Conversion6/1
  D-1LPF/1 -> Bus Creator/7  "mtrif_v_bus"

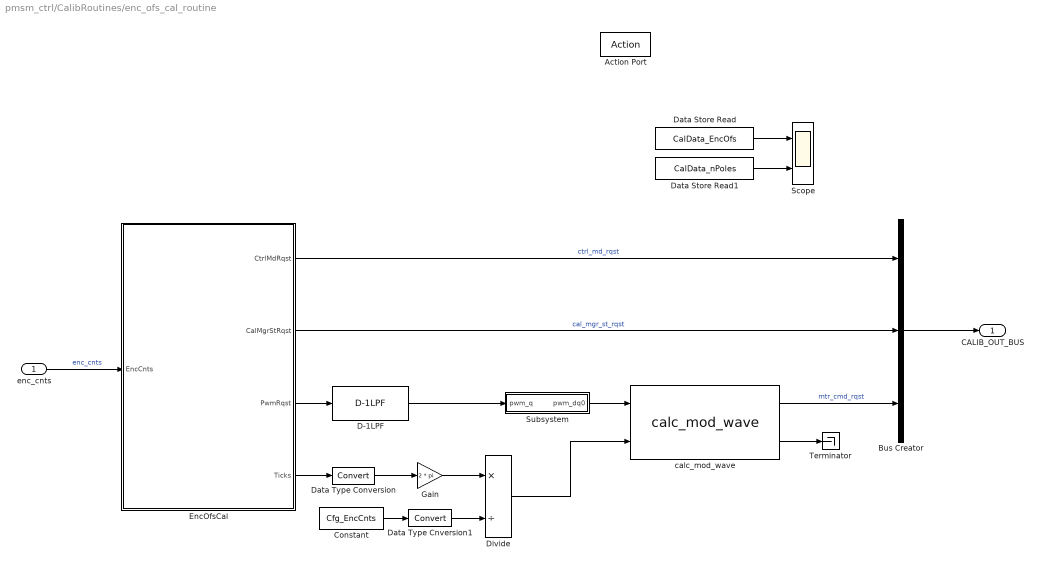
== system pmsm_ctrl/CalibRoutines/enc_ofs_cal_routine ==
  enc_cnts : Inport
  Action Port : ActionPort  InitializeStates=reset  ActionType=case
  Bus Creator : BusCreator  Inputs=3  OutDataTypeStr=Bus: Calib_OutType  NonVirtualBus=on
  Constant : Constant  Value=Cfg_EncCnts
  D-1LPF : ctrl_lib/D-1LPF  k_filt=0.9615
  Data Store Read : DataStoreRead  DataStoreName=CalData_EncOfs
  Data Store Read1 : DataStoreRead  DataStoreName=CalData_nPoles
  Data Type Cnversion1 : DataTypeConversion
  Data Type Conversion : DataTypeConversion
  Divide : Product  Inputs=*/
  EncOfsCal : Stateflow chart  TreatAsAtomicUnit=on
  Gain : Gain  Gain=2 * pi
      settings: AttributesFormatString=%<Gain>
  Scope : Scope  NumInputPorts=2
  Subsystem : Subsystem
  Terminator : Terminator
  calc_mod_wave : ctrl_lib/calc_mod_wave
  CALIB_OUT_BUS : Outport  OutDataTypeStr=Bus: Calib_OutType
  wires:
  enc_cnts/1 -> EncOfsCal/1(EncCnts)  "enc_cnts"
  Bus Creator/1 -> CALIB_OUT_BUS/1
  EncOfsCal/2(CalMgrStRqst) -> Bus Creator/2  "cal_mgr_st_rqst"
  EncOfsCal/1(CtrlMdRqst) -> Bus Creator/1  "ctrl_md_rqst"
  calc_mod_wave/1 -> Bus Creator/3  "mtr_cmd_rqst"
  Data Store Read/1 -> Scope/1
  EncOfsCal/3(PwmRqst) -> D-1LPF/1
  Subsystem/1(pwm_dq0) -> calc_mod_wave/1
  EncOfsCal/4(Ticks) -> Data Type Conversion/1
  calc_mod_wave/2 -> Terminator/1
  D-1LPF/1 -> Subsystem/1(pwm_q)
  Data Store Read1/1 -> Scope/2
  Divide/1 -> calc_mod_wave/2
  Data Type Conversion/1 -> Gain/1
  Gain/1 -> Divide/1
  Constant/1 -> Data Type Cnversion1/1
  Data Type Cnversion1/1 -> Divide/2

== system pmsm_ctrl/CalibRoutines/mtr_ifbk_ofs_ident ==
  mtr_ifbk_abc : Inport
  Action Port : ActionPort  InitializeStates=reset  ActionType=case
  Bus Creator : BusCreator  Inputs=3  OutDataTypeStr=Bus: Calib_OutType  NonVirtualBus=on
  Data Store Read : DataStoreRead  DataStoreName=CalData_IfbkOfs_Abc
  Display : Display
  ResIdCal : Stateflow chart  TreatAsAtomicUnit=on
  pwm_abc : Subsystem
  CALIB_OUT_BUS : Outport  OutDataTypeStr=Bus: Calib_OutType
  wires:
  pwm_abc/1(pwm_abc) -> Bus Creator/3  "mtr_cmd_rqst"
  ResIdCal/3(PwmRqst) -> pwm_abc/1(pwm_a)  "pwm_a"
  Bus Creator/1 -> CALIB_OUT_BUS/1
  mtr_ifbk_abc/1 -> ResIdCal/1(MtrIfbk)
  ResIdCal/2(CalMgrStRqst) -> Bus Creator/2  "cal_mgr_st_rqst"
  ResIdCal/1(CtrlMdRqst) -> Bus Creator/1  "ctrl_md_rqst"
  Data Store Read/1 -> Display/1

== system pmsm_ctrl/CalibRoutines/mtr_ind_ident ==
  mtr_ifbk_abc : Inport
  Action Port : ActionPort  InitializeStates=reset  ActionType=case
  Bus Creator : BusCreator  Inputs=3  OutDataTypeStr=Bus: Calib_OutType  NonVirtualBus=on
  Data Store Read : DataStoreRead  DataStoreName=CalData_L
  Display : Display
  IndIdCal : Stateflow chart  TreatAsAtomicUnit=on
  Selector : Selector  InputPortWidth=3  IndexOptions=Index vector (dialog)  Indices=[1]  OutputSizes=1
  calc_dc : Subsystem
  CALIB_OUT_BUS : Outport  OutDataTypeStr=Bus: Calib_OutType
  wires:
  Data Store Read/1 -> Display/1
  calc_dc/1(pwm_dc) -> Bus Creator/3  "mtr_cmd_rqst"
  IndIdCal/3(PwmRqst) -> calc_dc/1(pwm_a)  "pwm_a"
  Bus Creator/1 -> CALIB_OUT_BUS/1
  Selector/1 -> IndIdCal/1(MtrIfbk)  "mtr_ifbk"
  IndIdCal/2(CalMgrStRqst) -> Bus Creator/2  "cal_mgr_st_rqst"
  mtr_ifbk_abc/1 -> Selector/1
  IndIdCal/1(CtrlMdRqst) -> Bus Creator/1  "ctrl_md_rqst"

== system pmsm_ctrl/CalibRoutines/mtr_res_ident ==
  mtr_ifbk_abc : Inport
  Action Port : ActionPort  InitializeStates=reset  ActionType=case
  Bus Creator : BusCreator  Inputs=3  OutDataTypeStr=Bus: Calib_OutType  NonVirtualBus=on
  Data Store Read : DataStoreRead  DataStoreName=CalData_Res
  Display : Display
  ResIdCal : Stateflow chart  TreatAsAtomicUnit=on
  Selector : Selector  InputPortWidth=3  IndexOptions=Index vector (dialog)  Indices=[1]  OutputSizes=1
  calc_dc : Subsystem
  CALIB_OUT_BUS : Outport  OutDataTypeStr=Bus: Calib_OutType
  wires:
  ResIdCal/1(CtrlMdRqst) -> Bus Creator/1  "ctrl_md_rqst"
  mtr_ifbk_abc/1 -> Selector/1
  ResIdCal/2(CalMgrStRqst) -> Bus Creator/2  "cal_mgr_st_rqst"
  Selector/1 -> ResIdCal/1(MtrIfbk)
  Bus Creator/1 -> CALIB_OUT_BUS/1
  ResIdCal/3(PwmRqst) -> calc_dc/1(pwm_a)  "pwm_a"
  calc_dc/1(pwm_dc) -> Bus Creator/3  "mtr_cmd_rqst"
  Data Store Read/1 -> Display/1

== system pmsm_ctrl/CalibRoutines/not_active ==
  Action Port : ActionPort  InitializeStates=reset  ActionType=case
  Bus Creator : BusCreator  Inputs=3  OutDataTypeStr=Bus: Calib_OutType  NonVirtualBus=on
  Zero : Constant  Value=[0., 0., 0.]  OutDataTypeStr=single
  Zero1 : Constant  Value=CalMgrSt_T.ST_DONE
  Zero2 : Constant  Value=MtrCtrlMd_T.CTRL_MD_OFF
  CALIB_OUT_BUS : Outport  OutDataTypeStr=Bus: Calib_OutType
  wires:
  Zero2/1 -> Bus Creator/1  "ctrl_md_rqst"
  Zero1/1 -> Bus Creator/2  "cal_mgr_st_rqst"
  Bus Creator/1 -> CALIB_OUT_BUS/1
  Zero/1 -> Bus Creator/3  "mtr_cmd_rqst"

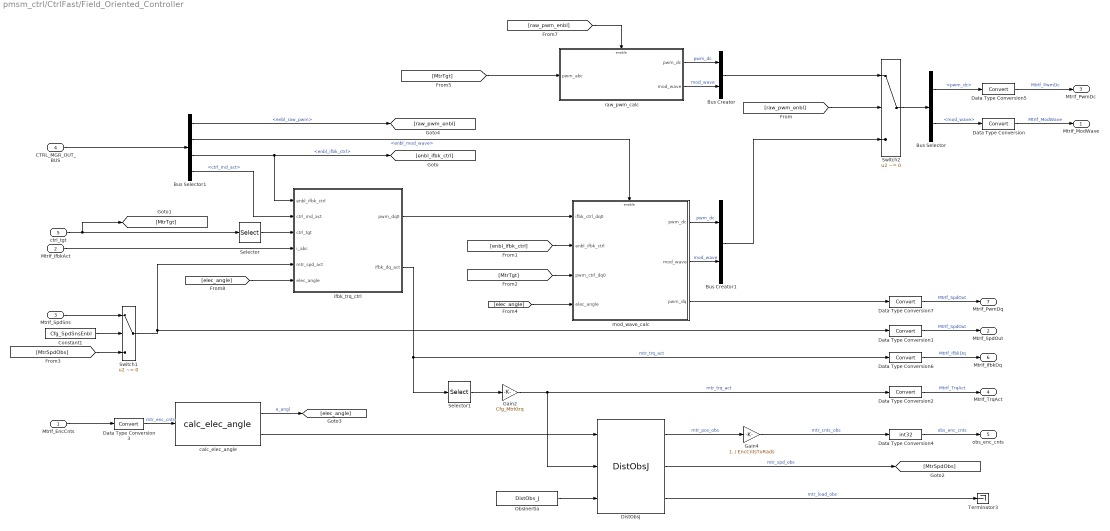
== system pmsm_ctrl/CtrlFast/Field_Oriented_Controller ==
  MtrIf_EncCnts : Inport
  MtrIf_IfbkAct : Inport  Port=2
  MtrIf_SpdSns : Inport  Port=3
  CTRL_MGR_OUT_BUS : Inport  Port=4
  ctrl_tgt : Inport  Port=5
  Bus Creator : BusCreator  Inputs=2
  Bus Creator1 : BusCreator  Inputs=2
  Bus Selector : BusSelector  OutputSignals=pwm_dc,mod_wave
  Bus Selector1 : BusSelector  OutputSignals=enbl_ctrl_flags.enbl_raw_pwm,enbl_ctrl_flags.enbl_mod_wave,enbl_ctrl_flags.enbl_ifbk_ctrl,ctrl_md_act
  Constant1 : Constant  Value=Cfg_SpdSnsEnbl
  Data Type Conversion{,1..3,5..7} (7 alike) : DataTypeConversion
  Data Type Conversion4 : DataTypeConversion  OutDataTypeStr=int32
  DistObsJ : adrc_lib/DistObsJ  ts=TsFast  k1=DistObs_K1  k2=DistObs_K2  k3=DistObs_K3
  Gain2 : Gain  Gain=Cfg_MtrKtrq  OutDataTypeStr=Inherit: Same as input
      settings: AttributesFormatString=%<Gain>
  Gain4 : Gain  Gain=1. / EncCntsToRads  OutDataTypeStr=Inherit: Inherit via back propagation
      settings: AttributesFormatString=%<Gain>
  ObsInertia : Constant  Value=DistObs_J
  Selector : Selector  InputPortWidth=3  IndexOptions=Index vector (dialog)  Indices=[1]  OutputSizes=1
  Selector1 : Selector  InputPortWidth=2  IndexOptions=Index vector (dialog)  Indices=[2]  OutputSizes=1
  Switch1 : Switch  Criteria=u2 ~= 0
      settings: AttributesFormatString=%<Criteria>
  Switch2 : Switch  Criteria=u2 ~= 0
      settings: AttributesFormatString=%<Criteria>
  Terminator3 : Terminator
  calc_elec_angle : ctrl_lib/calc_elec_angle  n_poles=Cfg_PolePairs  enc_cnts_int=Cfg_EncCnts
  ifbk_trq_ctrl : Subsystem
  mod_wave_calc : Subsystem
  raw_pwm_calc : Subsystem
  MtrIf_ModWave : Outport  InitialOutput=0
  MtrIf_SpdOut : Outport  Port=2  InitialOutput=0
  MtrIf_PwmDc : Outport  Port=3  InitialOutput=0
  MtrIf_TrqAct : Outport  Port=4  InitialOutput=0
  obs_enc_cnts : Outport  Port=5  InitialOutput=0
  MtrIf_IfbkDq : Outport  Port=6  InitialOutput=0
  MtrIf_PwmDq : Outport  Port=7  InitialOutput=0
  wires:
  Data Type Conversion2/1 -> MtrIf_TrqAct/1  "MtrIf_TrqAct"
  DistObsJ/2 -> [MtrSpdObs]  "mtr_spd_obs"
  Gain4/1 -> Data Type Conversion4/1  "mtr_cnts_obs"
  Data Type Conversion1/1 -> MtrIf_SpdOut/1  "MtrIf_SpdOut"
  MtrIf_EncCnts/1 -> Data Type Conversion3/1
  ctrl_tgt/1 -> Selector/1, [MtrTgt]
  ObsInertia/1 -> DistObsJ/3
  Data Type Conversion4/1 -> obs_enc_cnts/1  "obs_enc_cnts"
  MtrIf_SpdSns/1 -> Switch1/1
  Data Type Conversion3/1 -> calc_elec_angle/1  "mtr_enc_cnts"
  calc_elec_angle/1 -> [elec_angle]  "e_angl"
  Constant1/1 -> Switch1/2
  MtrIf_IfbkAct/1 -> ifbk_trq_ctrl/4(i_abc)
  Data Type Conversion/1 -> MtrIf_ModWave/1  "MtrIf_ModWave"
  Data Type Conversion5/1 -> MtrIf_PwmDc/1  "MtrIf_PwmDc"
  calc_elec_angle/2 -> DistObsJ/1
  Gain2/1 -> Data Type Conversion2/1, DistObsJ/2  "mtr_trq_act"
  Switch1/1 -> ifbk_trq_ctrl/5(mtr_spd_act), Data Type Conversion1/1
  DistObsJ/3 -> Terminator3/1  "mtr_load_obs"
  [MtrSpdObs] -> Switch1/3
  Bus Selector1/3 -> [enbl_ifbk_ctrl], ifbk_trq_ctrl/1(enbl_ifbk_ctrl)  "<enbl_ifbk_ctrl>"
  Bus Selector1/2 -> mod_wave_calc/Enable  "<enbl_mod_wave>"
  [enbl_ifbk_ctrl] -> mod_wave_calc/2(enbl_ifbk_ctrl)
  [MtrTgt] -> mod_wave_calc/3(pwm_ctrl_dq0)
  [elec_angle] -> mod_wave_calc/4(elec_angle)
  [MtrTgt] -> raw_pwm_calc/1(pwm_abc)
  Bus Selector1/1 -> [raw_pwm_enbl]  "<enbl_raw_pwm>"
  [raw_pwm_enbl] -> Switch2/2
  [raw_pwm_enbl] -> raw_pwm_calc/Enable
  Switch2/1 -> Bus Selector/1
  Bus Selector/2 -> Data Type Conversion/1  "<mod_wave>"
  [elec_angle] -> ifbk_trq_ctrl/6(elec_angle)
  raw_pwm_calc/1(pwm_dc) -> Bus Creator/1  "pwm_dc"
  raw_pwm_calc/2(mod_wave) -> Bus Creator/2  "mod_wave"
  Bus Creator/1 -> Switch2/1
  mod_wave_calc/1(pwm_dc) -> Bus Creator1/1  "pwm_dc"
  mod_wave_calc/2(mod_wave) -> Bus Creator1/2  "mod_wave"
  Bus Creator1/1 -> Switch2/3
  Bus Selector/1 -> Data Type Conversion5/1  "<pwm_dc>"
  CTRL_MGR_OUT_BUS/1 -> Bus Selector1/1
  Selector/1 -> ifbk_trq_ctrl/3(ctrl_tgt)
  Bus Selector1/4 -> ifbk_trq_ctrl/2(ctrl_md_act)  "<ctrl_md_act>"
  ifbk_trq_ctrl/2(ifbk_dq_act) -> Data Type Conversion6/1, Selector1/1  "mtr_trq_act"
  Data Type Conversion6/1 -> MtrIf_IfbkDq/1  "MtrIf_IfbkDq"
  Selector1/1 -> Gain2/1
  Data Type Conversion7/1 -> MtrIf_PwmDq/1  "MtrIf_SpdOut"
  ifbk_trq_ctrl/1(pwm_dq0) -> mod_wave_calc/1(ifbk_ctrl_dq0)
  mod_wave_calc/3(pwm_dq) -> Data Type Conversion7/1
  DistObsJ/1 -> Gain4/1  "mtr_pos_obs"

== system pmsm_ctrl/CtrlFast/det_ctrl_tgt ==
  CTRL_MGR_OUT_BUS : Inport
  MOTN_CTRL_OUT_BUS : Inport  Port=2
  Bus Selector1 : BusSelector  OutputSignals=motn_ctrl_cmd
  Bus Selector2 : BusSelector  OutputSignals=ctrl_tgt,enbl_ctrl_flags.enbl_spd_ctrl,enbl_ctrl_flags.enbl_pos_ctrl
  Gain : Gain  Gain=[1., 0., 0.]
  Logical Operator : Logic  Operator=OR  AllPortsSameDT=off  OutDataTypeStr=boolean
  Logical Operator1 : Logic  Operator=NOT  AllPortsSameDT=off  OutDataTypeStr=boolean
  Switch : Switch  Criteria=u2 ~= 0
  ctrl_tgt : Outport
  wires:
  Logical Operator/1 -> Logical Operator1/1  "motn_ctrl_enbl"
  Bus Selector2/2 -> Logical Operator/1  "<enbl_spd_ctrl>"
  Bus Selector2/1 -> Switch/1  "<ctrl_tgt>"
  Bus Selector1/1 -> Gain/1  "<motn_ctrl_cmd>"
  Bus Selector2/3 -> Logical Operator/2  "<enbl_pos_ctrl>"
  CTRL_MGR_OUT_BUS/1 -> Bus Selector2/1
  MOTN_CTRL_OUT_BUS/1 -> Bus Selector1/1
  Logical Operator1/1 -> Switch/2
  Switch/1 -> ctrl_tgt/1
  Gain/1 -> Switch/3

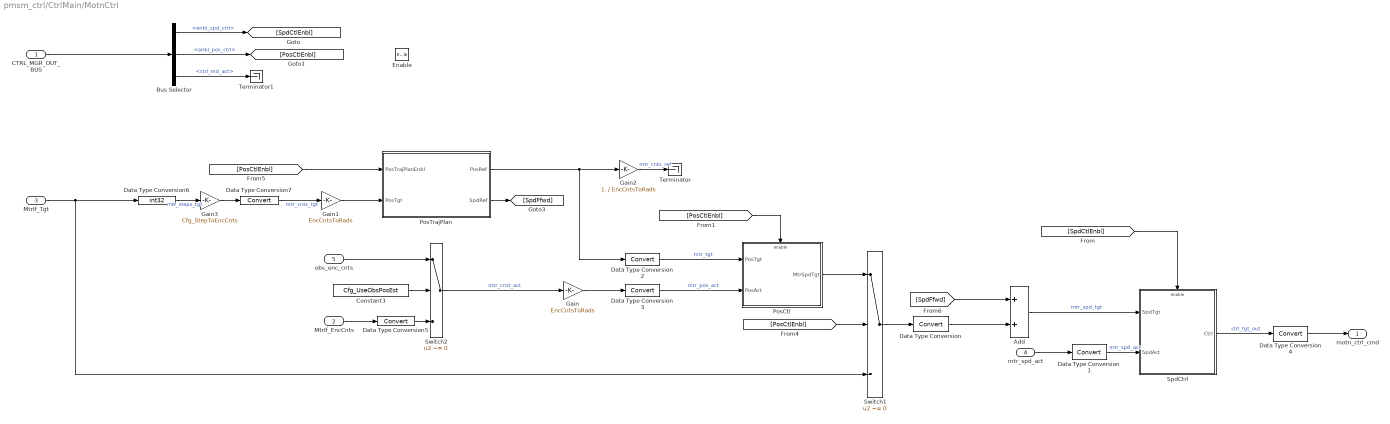
== system pmsm_ctrl/CtrlMain/MotnCtrl ==
  CTRL_MGR_OUT_BUS : Inport
  MtrIf_EncCnts : Inport  Port=2
  MtrIf_Tgt : Inport  Port=3
  mtr_spd_act : Inport  Port=4
  obs_enc_cnts : Inport  Port=5
  Enable : EnablePort  StatesWhenEnabling=reset
  Add : Sum
  Bus Selector : BusSelector  OutputSignals=enbl_ctrl_flags.enbl_spd_ctrl,enbl_ctrl_flags.enbl_pos_ctrl,ctrl_md_act
  Constant3 : Constant  Value=Cfg_UseObsPosEst
  Data Type Conversion{,1..5,7} (7 alike) : DataTypeConversion
  Data Type Conversion6 : DataTypeConversion  OutDataTypeStr=int32
  Gain : Gain  Gain=EncCntsToRads
      settings: AttributesFormatString=%<Gain>
  Gain1 : Gain  Gain=EncCntsToRads
      settings: AttributesFormatString=%<Gain>
  Gain2 : Gain  Gain=1. / EncCntsToRads
      settings: AttributesFormatString=%<Gain>
  Gain3 : Gain  Gain=Cfg_StepToEncCnts  ParamDataTypeStr=Inherit: Inherit from 'Gain'  OutDataTypeStr=Inherit: Same as input
      settings: AttributesFormatString=%<Gain>
  PosCtl : Subsystem
  PosTrajPlan : Subsystem
  SpdCtrl : Subsystem
  Switch1 : Switch  Criteria=u2 ~= 0  Threshold=MtrCtrlMd.SpdCtrlMd
      settings: AttributesFormatString=%<Criteria>
  Switch2 : Switch  Criteria=u2 ~= 0
  Terminator : Terminator
  Terminator1 : Terminator
  motn_ctrl_cmd : Outport  InitialOutput=0
  wires:
  PosCtl/1(MtrSpdTgt) -> Switch1/1
  Switch1/1 -> Data Type Conversion/1
  MtrIf_EncCnts/1 -> Data Type Conversion5/1
  Data Type Conversion3/1 -> PosCtl/2(PosAct)  "mtr_pos_act"
  [PosCtlEnbl] -> Switch1/2
  PosTrajPlan/2(SpdRef) -> [SpdFfwd]
  MtrIf_Tgt/1 -> Data Type Conversion6/1, Switch1/3
  Constant3/1 -> Switch2/2
  Data Type Conversion/1 -> Add/2
  Gain/1 -> Data Type Conversion3/1
  obs_enc_cnts/1 -> Switch2/1
  Data Type Conversion6/1 -> Gain3/1  "mtr_steps_tgt"
  Data Type Conversion5/1 -> Switch2/3
  Bus Selector/2 -> [PosCtlEnbl]  "<enbl_pos_ctrl>"
  PosTrajPlan/1(PosRef) -> Gain2/1, Data Type Conversion2/1
  Add/1 -> SpdCtrl/1(SpdTgt)  "mtr_spd_tgt"
  [PosCtlEnbl] -> PosCtl/Enable
  [PosCtlEnbl] -> PosTrajPlan/1(PosTrajPlanEnbl)
  Data Type Conversion2/1 -> PosCtl/1(PosTgt)  "mtr_tgt"
  Gain1/1 -> PosTrajPlan/2(PosTgt)
  [SpdFfwd] -> Add/1
  Gain2/1 -> Terminator/1  "mtr_cnts_ref"
  Gain3/1 -> Data Type Conversion7/1
  Data Type Conversion7/1 -> Gain1/1  "mtr_cnts_tgt"
  [SpdCtlEnbl] -> SpdCtrl/Enable
  Switch2/1 -> Gain/1  "mtr_cnst_act"
  mtr_spd_act/1 -> Data Type Conversion1/1
  Bus Selector/1 -> [SpdCtlEnbl]  "<enbl_spd_ctrl>"
  Data Type Conversion1/1 -> SpdCtrl/2(SpdAct)  "mtr_spd_act"
  SpdCtrl/1(Ctrl) -> Data Type Conversion4/1  "ctrl_tgt_out"
  Data Type Conversion4/1 -> motn_ctrl_cmd/1
  CTRL_MGR_OUT_BUS/1 -> Bus Selector/1
  Bus Selector/3 -> Terminator1/1  "<ctrl_md_act>"

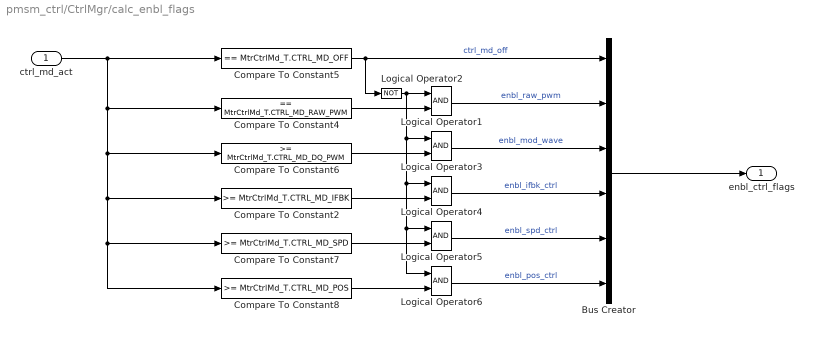
== system pmsm_ctrl/CtrlMgr/calc_enbl_flags ==
  ctrl_md_act : Inport
  Bus Creator : BusCreator  Inputs=6
  Compare To Constant2 : simulink/Logic and Bit Operations/Compare To Constant  relop=>=  const=MtrCtrlMd_T.CTRL_MD_IFBK  OutDataTypeStr=boolean
  Compare To Constant4 : simulink/Logic and Bit Operations/Compare To Constant  relop===  const=MtrCtrlMd_T.CTRL_MD_RAW_PWM  OutDataTypeStr=boolean
  Compare To Constant5 : simulink/Logic and Bit Operations/Compare To Constant  relop===  const=MtrCtrlMd_T.CTRL_MD_OFF  OutDataTypeStr=boolean
  Compare To Constant6 : simulink/Logic and Bit Operations/Compare To Constant  relop=>=  const=MtrCtrlMd_T.CTRL_MD_DQ_PWM  OutDataTypeStr=boolean
  Compare To Constant7 : simulink/Logic and Bit Operations/Compare To Constant  relop=>=  const=MtrCtrlMd_T.CTRL_MD_SPD  OutDataTypeStr=boolean
  Compare To Constant8 : simulink/Logic and Bit Operations/Compare To Constant  relop=>=  const=MtrCtrlMd_T.CTRL_MD_POS  OutDataTypeStr=boolean
  Logical Operator{1,3..6} (5 alike) : Logic  AllPortsSameDT=off  OutDataTypeStr=boolean
  Logical Operator2 : Logic  Operator=NOT  AllPortsSameDT=off  OutDataTypeStr=boolean
  enbl_ctrl_flags : Outport
  wires:
  Compare To Constant8/1 -> Logical Operator6/2
  Compare To Constant2/1 -> Logical Operator4/2
  Logical Operator1/1 -> Bus Creator/2  "enbl_raw_pwm"
  Compare To Constant6/1 -> Logical Operator3/2
  Logical Operator5/1 -> Bus Creator/5  "enbl_spd_ctrl"
  Compare To Constant4/1 -> Logical Operator1/2
  Bus Creator/1 -> enbl_ctrl_flags/1
  Logical Operator2/1 -> Logical Operator6/1, Logical Operator5/1, Logical Operator4/1, Logical Operator3/1, Logical Operator1/1
  Logical Operator6/1 -> Bus Creator/6  "enbl_pos_ctrl"
  Compare To Constant7/1 -> Logical Operator5/2
  Logical Operator3/1 -> Bus Creator/3  "enbl_mod_wave"
  Logical Operator4/1 -> Bus Creator/4  "enbl_ifbk_ctrl"
  Compare To Constant5/1 -> Logical Operator2/1, Bus Creator/1  "ctrl_md_off"
  ctrl_md_act/1 -> Compare To Constant8/1, Compare To Constant7/1, Compare To Constant2/1, Compare To Constant6/1, Compare To Constant4/1, Compare To Constant5/1

== system pmsm_ctrl/SetInputs/enc_ofs_comp ==
  enc_cnts_raw : Inport
  "enc_ofs " : Inport  Port=2
  Subtract : Sum  Inputs=+-
  enc_cnts : Outport
  wires:
  enc_cnts_raw/1 -> Subtract/1
  "enc_ofs "/1 -> Subtract/2
  Subtract/1 -> enc_cnts/1

== system pmsm_ctrl/SetInputs/ifbk_ofs_comp ==
  ifbk_raw : Inport
  "ifbk_ofs " : Inport  Port=2
  Subtract : Sum  Inputs=+-
  ifbk : Outport
  wires:
  Subtract/1 -> ifbk/1
  "ifbk_ofs "/1 -> Subtract/2
  ifbk_raw/1 -> Subtract/1

== system pmsm_ctrl/CalibRoutines/enc_ofs_cal_routine/Subsystem ==
  pwm_q : Inport
  Constant : Constant  Value=0.  OutDataTypeStr=single
  Mux : Mux  Inputs=3
  pwm_dq0 : Outport
  wires:
  Mux/1 -> pwm_dq0/1
  pwm_q/1 -> Mux/1
  Constant/1 -> Mux/3, Mux/2

== system pmsm_ctrl/CalibRoutines/mtr_ifbk_ofs_ident/ResIdCal/get_mtr_ifbk_avg ==
  mtr_ifbk_sum_abc : Inport  PortDimensions=3
  ncycles : Inport  Port=2
  call : TriggerPort  TriggerType=function-call  VariantControl=(inherit)  StatesWhenEnabling=reset
      settings: CopyFcn=Stateflow.SLINSF.SimulinkMan.removeBlockPreDeleteFcn  PreDeleteFcn=Stateflow.SLINSF.SimulinkMan.unsafePredeleteFcn
  Divide : Product  Inputs=*/
  Saturation : Saturate  UpperLimit=1e6  LowerLimit=1
  mtr_ifbk_avg_abc : Outport
  wires:
  mtr_ifbk_sum_abc/1 -> Divide/1
  Divide/1 -> mtr_ifbk_avg_abc/1
  ncycles/1 -> Saturation/1
  Saturation/1 -> Divide/2

== system pmsm_ctrl/CalibRoutines/mtr_ifbk_ofs_ident/ResIdCal/get_mtr_ifbk_sum ==
  mtr_ifbk_abc : Inport  PortDimensions=3
  call : TriggerPort  TriggerType=function-call  VariantControl=(inherit)  StatesWhenEnabling=reset
      settings: CopyFcn=Stateflow.SLINSF.SimulinkMan.removeBlockPreDeleteFcn  PreDeleteFcn=Stateflow.SLINSF.SimulinkMan.unsafePredeleteFcn
  Add : Sum
  Unit Delay : UnitDelay  SampleTime=-1
  mtr_ifbk_sum_abc : Outport
  wires:
  mtr_ifbk_abc/1 -> Add/1
  Unit Delay/1 -> Add/2
  Add/1 -> mtr_ifbk_sum_abc/1, Unit Delay/1

== system pmsm_ctrl/CalibRoutines/mtr_ifbk_ofs_ident/pwm_abc ==
  pwm_a : Inport
  Mux : Mux  Inputs=3
  Zero : Constant  Value=0  OutDataTypeStr=single
  pwm_abc : Outport
  wires:
  Mux/1 -> pwm_abc/1
  pwm_a/1 -> Mux/1
  Zero/1 -> Mux/2, Mux/3

== system pmsm_ctrl/CalibRoutines/mtr_ind_ident/calc_dc ==
  pwm_a : Inport
  Mux : Mux  Inputs=3
  Zero : Constant  Value=0  OutDataTypeStr=single
  calc_pwm_dc : ctrl_lib/calc_pwm_dc
  pwm_dc : Outport
  wires:
  calc_pwm_dc/1 -> pwm_dc/1
  Mux/1 -> calc_pwm_dc/1
  pwm_a/1 -> Mux/1
  Zero/1 -> Mux/2, Mux/3

== system pmsm_ctrl/CalibRoutines/mtr_res_ident/calc_dc ==
  pwm_a : Inport
  Mux : Mux  Inputs=3
  Zero : Constant  Value=0  OutDataTypeStr=single
  calc_pwm_dc : ctrl_lib/calc_pwm_dc
  pwm_dc : Outport
  wires:
  Zero/1 -> Mux/3, Mux/2
  pwm_a/1 -> Mux/1
  Mux/1 -> calc_pwm_dc/1
  calc_pwm_dc/1 -> pwm_dc/1

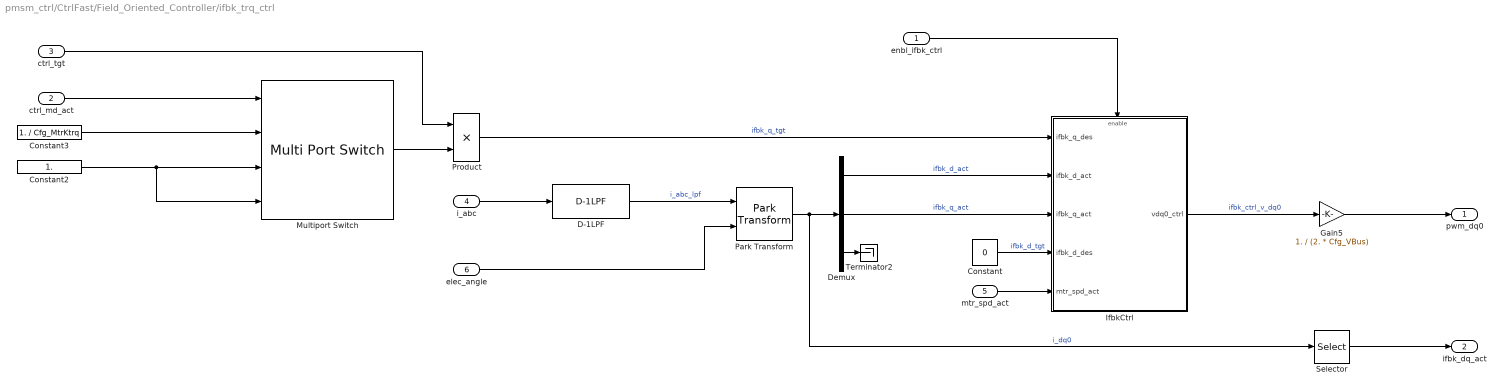
== system pmsm_ctrl/CtrlFast/Field_Oriented_Controller/ifbk_trq_ctrl ==
  enbl_ifbk_ctrl : Inport
  ctrl_md_act : Inport  Port=2
  ctrl_tgt : Inport  Port=3
  i_abc : Inport  Port=4
  mtr_spd_act : Inport  Port=5
  elec_angle : Inport  Port=6
  Constant : Constant  Value=0  OutDataTypeStr=Inherit: Inherit via back propagation
  Constant2 : Constant  Value=1.  OutDataTypeStr=Inherit: Inherit via back propagation
  Constant3 : Constant  Value=1. / Cfg_MtrKtrq  OutDataTypeStr=Inherit: Inherit via back propagation
  D-1LPF : ctrl_lib/D-1LPF  k_filt=1e-4/ (1e-4 + TsFast)
  Demux : Demux  Outputs=3
  Gain5 : Gain  Gain=1. / (2. * Cfg_VBus)
      settings: AttributesFormatString=%<Gain>
  IfbkCtrl : Subsystem
  Multiport Switch : MultiPortSwitch  DataPortOrder=Specify indices  Inputs=2  DataPortIndices={MtrCtrlMd_T.CTRL_MD_TRQ, MtrCtrlMd_T.CTRL_MD_IFBK}  DataPortForDefault=Additional data port  DiagnosticForDefault=Warning
  Park Transform : peTransforms/Park Transform  AxisAlignment=D-axis  PowerInvariant=off
  Product : Product
  Selector : Selector  InputPortWidth=3  IndexOptions=Index vector (dialog)  Indices=[1 2]  OutputSizes=1
  Terminator2 : Terminator
  pwm_dq0 : Outport
  ifbk_dq_act : Outport  Port=2
  wires:
  Demux/1 -> IfbkCtrl/2(ifbk_d_act)  "ifbk_d_act"
  i_abc/1 -> D-1LPF/1
  Gain5/1 -> pwm_dq0/1
  elec_angle/1 -> Park Transform/2
  Demux/3 -> Terminator2/1
  D-1LPF/1 -> Park Transform/1  "i_abc_lpf"
  Constant/1 -> IfbkCtrl/4(ifbk_d_des)  "ifbk_d_tgt"
  IfbkCtrl/1(vdq0_ctrl) -> Gain5/1  "ifbk_ctrl_v_dq0"
  Demux/2 -> IfbkCtrl/3(ifbk_q_act)  "ifbk_q_act"
  Product/1 -> IfbkCtrl/1(ifbk_q_des)  "ifbk_q_tgt"
  mtr_spd_act/1 -> IfbkCtrl/5(mtr_spd_act)
  Park Transform/1 -> Selector/1, Demux/1  "i_dq0"
  Multiport Switch/1 -> Product/2
  ctrl_tgt/1 -> Product/1
  Constant2/1 -> Multiport Switch/4, Multiport Switch/3
  Constant3/1 -> Multiport Switch/2
  ctrl_md_act/1 -> Multiport Switch/1
  Selector/1 -> ifbk_dq_act/1
  enbl_ifbk_ctrl/1 -> IfbkCtrl/Enable

== system pmsm_ctrl/CtrlFast/Field_Oriented_Controller/mod_wave_calc ==
  ifbk_ctrl_dq0 : Inport
  enbl_ifbk_ctrl : Inport  Port=2
  pwm_ctrl_dq0 : Inport  Port=3
  elec_angle : Inport  Port=4
  Enable : EnablePort  StatesWhenEnabling=reset
  Saturation1 : Saturate  UpperLimit=1.  LowerLimit=-1.
      settings: AttributesFormatString=[%<LowerLimit>, %<UpperLimit>]
  Selector2 : Selector  InputPortWidth=3  IndexOptions=Index vector (dialog)  Indices=[1 2]  OutputSizes=1
  Switch : Switch  Criteria=u2 ~= 0
      settings: AttributesFormatString=%<Criteria>
  calc_mod_wave : ctrl_lib/calc_mod_wave
  pwm_dc : Outport
  mod_wave : Outport  Port=2
  pwm_dq : Outport  Port=3
  wires:
  pwm_ctrl_dq0/1 -> Switch/3
  Switch/1 -> Saturation1/1  "pwm_dq0"
  enbl_ifbk_ctrl/1 -> Switch/2
  Saturation1/1 -> Selector2/1, calc_mod_wave/1
  calc_mod_wave/2 -> mod_wave/1
  elec_angle/1 -> calc_mod_wave/2
  ifbk_ctrl_dq0/1 -> Switch/1
  calc_mod_wave/1 -> pwm_dc/1
  Selector2/1 -> pwm_dq/1

== system pmsm_ctrl/CtrlFast/Field_Oriented_Controller/raw_pwm_calc ==
  pwm_abc : Inport
  Enable : EnablePort  StatesWhenEnabling=reset
  Saturation : Saturate  UpperLimit=1.  LowerLimit=0.
  Scope : Scope  NumInputPorts=2
  Zero1 : Constant  Value=[0., 0., 0.]  OutDataTypeStr=Inherit: Inherit via back propagation
  raw_pwm_calc : ctrl_lib/calc_pwm_dc  Commented=through
  pwm_dc : Outport
  mod_wave : Outport  Port=2
  wires:
  Zero1/1 -> mod_wave/1
  pwm_abc/1 -> Saturation/1  "pwm_abc"
  Saturation/1 -> Scope/1, raw_pwm_calc/1
  raw_pwm_calc/1 -> Scope/2, pwm_dc/1

== system pmsm_ctrl/CtrlMain/MotnCtrl/PosCtl ==
  PosTgt : Inport
  PosAct : Inport  Port=2
  Enable : EnablePort  StatesWhenEnabling=reset
  PI-Ctrl : ctrl_lib/PI-Ctrl  ts=TsMain  PI_Kp=PosCtrl_Kp  PI_Ki=PosCtrl_Ki  max_lim=1000  min_lim=-1000
  MtrSpdTgt : Outport
  wires:
  PI-Ctrl/1 -> MtrSpdTgt/1  "MtrSpdTgt"
  PosTgt/1 -> PI-Ctrl/1
  PosAct/1 -> PI-Ctrl/2

== system pmsm_ctrl/CtrlMain/MotnCtrl/PosTrajPlan ==
  PosTrajPlanEnbl : Inport
  PosTgt : Inport  Port=2
  Constant : Constant  Value=Cfg_EnblTrajPlan
  Logical Operator : Logic  AllPortsSameDT=off  OutDataTypeStr=boolean
  PosTrackDiff : Subsystem  AncestorBlock=adrc_lib/TrackDiff  mask{ts=1e-3, h0=1e-3, r0=5e3}
      mask prompts: ts "Exeuction rate [s]:"
  Switch : Switch  Criteria=u2 ~= 0
      settings: AttributesFormatString=%<Criteria>
  PosRef : Outport
  SpdRef : Outport  Port=2
  wires:
  PosTrajPlanEnbl/1 -> Logical Operator/2
  PosTgt/1 -> [Tgt], PosTrackDiff/1(MtrTgt)
  PosTrackDiff/2(Grd) -> SpdRef/1  "traj_plan_grd"
  Switch/1 -> PosRef/1
  PosTrackDiff/1(Ref) -> Switch/1  "traj_plan_ref"
  [Enbl] -> Switch/2
  [Tgt] -> Switch/3
  Logical Operator/1 -> [Enbl], PosTrackDiff/Enable  "traj_plan_is_enbl"
  Constant/1 -> Logical Operator/1

== system pmsm_ctrl/CtrlMain/MotnCtrl/SpdCtrl ==
  SpdTgt : Inport
  SpdAct : Inport  Port=2
  Enable : EnablePort  StatesWhenEnabling=reset
  Constant1 : Constant  Value=Cfg_SpdCtrlBW * Cfg_MtrKf
  Constant3 : Constant  Value=Cfg_SpdCtrlBW * Cfg_MtrJm
  PI-Ctrl-Varying-Gains : ctrl_lib/PI-Ctrl-Varying-Gains  ts=TsFast  max_lim=10  min_lim=-10
  Saturation : Saturate  UpperLimit=10  LowerLimit=-10
  Ctrl : Outport
  wires:
  SpdAct/1 -> PI-Ctrl-Varying-Gains/2
  PI-Ctrl-Varying-Gains/1 -> Saturation/1
  Constant3/1 -> PI-Ctrl-Varying-Gains/3
  Constant1/1 -> PI-Ctrl-Varying-Gains/4
  Saturation/1 -> Ctrl/1
  SpdTgt/1 -> PI-Ctrl-Varying-Gains/1

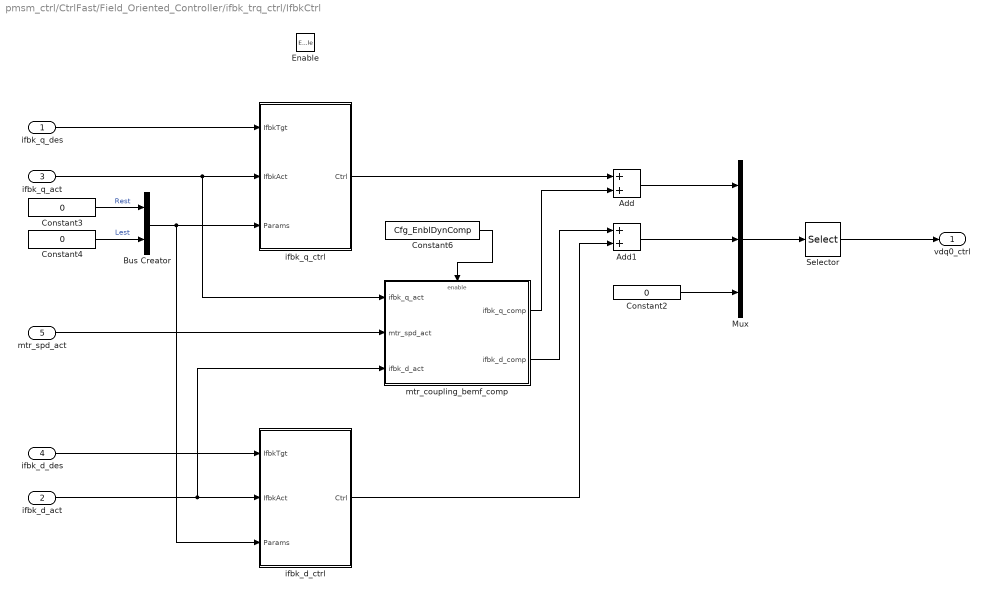
== system pmsm_ctrl/CtrlFast/Field_Oriented_Controller/ifbk_trq_ctrl/IfbkCtrl ==
  ifbk_q_des : Inport
  ifbk_d_act : Inport  Port=2
  ifbk_q_act : Inport  Port=3
  ifbk_d_des : Inport  Port=4
  mtr_spd_act : Inport  Port=5
  Enable : EnablePort  StatesWhenEnabling=reset
  Add : Sum
  Add1 : Sum
  Bus Creator : BusCreator  Inputs=2
  Constant2 : Constant  Value=0  OutDataTypeStr=Inherit: Inherit via back propagation
  Constant3 : Constant  Value=0  OutDataTypeStr=Inherit: Inherit via back propagation
  Constant4 : Constant  Value=0  OutDataTypeStr=Inherit: Inherit via back propagation
  Constant6 : Constant  Value=Cfg_EnblDynComp  OutDataTypeStr=boolean
  Mux : Mux  Inputs=3
  Selector : Selector  InputPortWidth=3  IndexOptions=Index vector (dialog)  Indices=[2 1 3]  OutputSizes=1
  ifbk_d_ctrl : Subsystem
  ifbk_q_ctrl : Subsystem
  mtr_coupling_bemf_comp : Subsystem
  vdq0_ctrl : Outport
  wires:
  Bus Creator/1 -> ifbk_q_ctrl/3(Params), ifbk_d_ctrl/3(Params)
  ifbk_q_des/1 -> ifbk_q_ctrl/1(IfbkTgt)
  ifbk_q_act/1 -> mtr_coupling_bemf_comp/1(ifbk_q_act), ifbk_q_ctrl/2(IfbkAct)
  ifbk_d_act/1 -> mtr_coupling_bemf_comp/3(ifbk_d_act), ifbk_d_ctrl/2(IfbkAct)
  ifbk_d_des/1 -> ifbk_d_ctrl/1(IfbkTgt)
  Constant3/1 -> Bus Creator/1  "Rest"
  Constant4/1 -> Bus Creator/2  "Lest"
  ifbk_q_ctrl/1(Ctrl) -> Add/1
  mtr_spd_act/1 -> mtr_coupling_bemf_comp/2(mtr_spd_act)
  mtr_coupling_bemf_comp/1(ifbk_q_comp) -> Add/2
  mtr_coupling_bemf_comp/2(ifbk_d_comp) -> Add1/1
  ifbk_d_ctrl/1(Ctrl) -> Add1/2
  Mux/1 -> Selector/1
  Add/1 -> Mux/1
  Add1/1 -> Mux/2
  Constant2/1 -> Mux/3
  Constant6/1 -> mtr_coupling_bemf_comp/Enable
  Selector/1 -> vdq0_ctrl/1

== system pmsm_ctrl/CtrlMain/MotnCtrl/PosTrajPlan/PosTrackDiff ==
  MtrTgt : Inport
  Enable : EnablePort  StatesWhenEnabling=reset
  Add : Sum  Inputs=-+
  Discrete-Time Integrator : DiscreteIntegrator  IntegratorMethod=Accumulation: Forward Euler  gainval=ts  SampleTime=-1  ICPrevOutput=DiscIntNeverNeededParam  ICPrevScaledInput=DiscIntNeverNeededParam
  Discrete-Time Integrator1 : DiscreteIntegrator  IntegratorMethod=Accumulation: Forward Euler  gainval=ts  SampleTime=-1  ICPrevOutput=DiscIntNeverNeededParam  ICPrevScaledInput=DiscIntNeverNeededParam
  fhan : adrc_lib/fhan  r0=r0  h0=h0
  Ref : Outport
  Grd : Outport  Port=2
  wires:
  MtrTgt/1 -> Add/1
  Add/1 -> fhan/1
  fhan/1 -> Discrete-Time Integrator/1
  Discrete-Time Integrator/1 -> Grd/1, fhan/2, Discrete-Time Integrator1/1
  Discrete-Time Integrator1/1 -> Add/2, Ref/1

== system pmsm_ctrl/CtrlFast/Field_Oriented_Controller/ifbk_trq_ctrl/IfbkCtrl/ifbk_d_ctrl ==
  IfbkTgt : Inport
  IfbkAct : Inport  Port=2
  Params : Inport  Port=3
  Bus Selector : BusSelector  OutputSignals=Lest,Rest
  Constant : Constant  Value=MtrParams.Ls * Cfg_IfbkCtrlBW
  Constant1 : Constant  Value=MtrParams.Rs * Cfg_IfbkCtrlBW
  Constant2 : Constant  Value=Cfg_AutoCalEnbl
  Constant3 : Constant  Value=Cfg_IfbkCtrlBW
  Demux : Demux  Outputs=2
  Mux : Mux  Inputs=2
  Mux1 : Mux  Inputs=2
  PI-Ctrl-Varying-Gains : ctrl_lib/PI-Ctrl-Varying-Gains  ts=TsFast  max_lim=12  min_lim=-12
  Product : Product
  Switch : Switch  Criteria=u2 ~= 0
  Ctrl : Outport
  wires:
  Constant3/1 -> Product/1
  Product/1 -> Switch/1
  Mux1/1 -> Switch/3
  Constant2/1 -> Switch/2
  Mux/1 -> Product/2
  Switch/1 -> Demux/1
  Constant1/1 -> Mux1/2
  Constant/1 -> Mux1/1
  Demux/2 -> PI-Ctrl-Varying-Gains/4
  Demux/1 -> PI-Ctrl-Varying-Gains/3
  Bus Selector/1 -> Mux/1  "<Lest>"
  Bus Selector/2 -> Mux/2  "<Rest>"
  Params/1 -> Bus Selector/1
  PI-Ctrl-Varying-Gains/1 -> Ctrl/1  "ifbk_d_ctrl_out"
  IfbkAct/1 -> PI-Ctrl-Varying-Gains/2
  IfbkTgt/1 -> PI-Ctrl-Varying-Gains/1
